simulink model "kalman"  (R2017a)
settings: Solver=VariableStepAuto  StartTime=0  StopTime=65  RelTol=1e-5
undefined symbols (not defined in the file): Discrete, Time
libraries: dspfdesign x3, ctrlSharedLib x1
settings Model: Creator=13291  LastModifiedBy=13291
settings DataIOCC: ExternalInput=[t, u, c1, c2]  LoadExternalInput=on

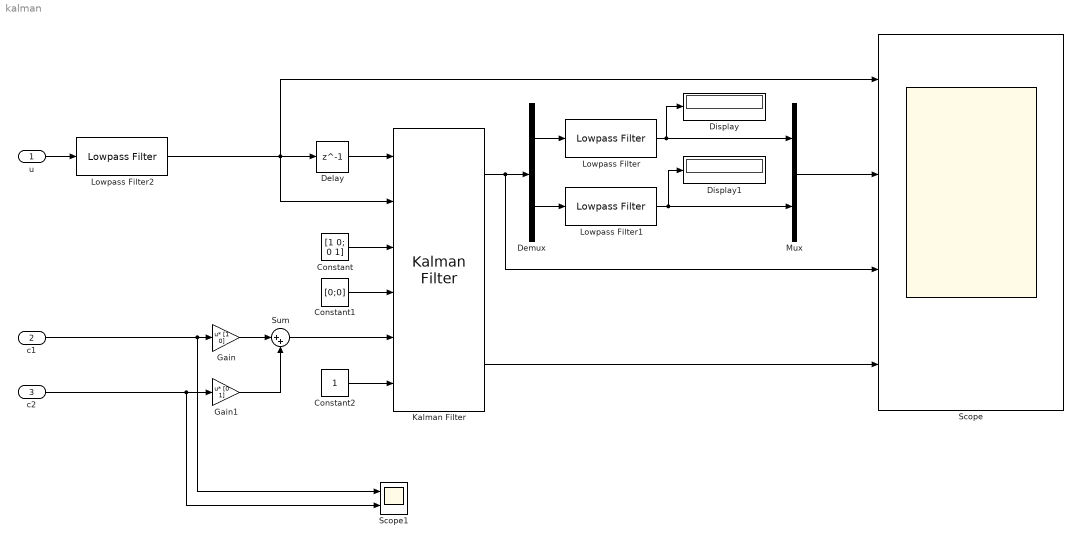
== system kalman ==
  u : Inport  PortDimensions=1  SampleTime=0.002
  c1 : Inport  Port=2  PortDimensions=1  SampleTime=0.002
  c2 : Inport  Port=3  PortDimensions=1  SampleTime=0.002
  Constant : Constant  Value=[1 0; 0 1]  VectorParams1D=off
  Constant1 : Constant  Value=[0;0]  VectorParams1D=off  LockScale=on
  Constant2 : Constant
  Delay : Delay  DelayLength=1
  Demux : Demux  Outputs=2
  Display : Display
  Display1 : Display
  Gain : Gain  Gain=[1 0]  Multiplication=Matrix(u*K)
  Gain1 : Gain  Gain=[0 1]  Multiplication=Matrix(u*K)
  Kalman Filter : ctrlSharedLib/Kalman Filter  TimeDomain=Discrete-Time  UseCurrentEstimator=on  ModelSource=Input port  ModelSourceVariable=ss(0.95,1,1,0,1)  A=0.95  B=1  C=1  D=0  NumberOfStates=2  NumberOfInputs=1  NumberOfOutputs=1  InitialEstimateSource=Dialog  X0=0  P0=10  UseK=off  UseGH=off  NumberOfProcessNoiseInputs=1  G=1  TimeInvariantG=on  H=0  TimeInvariantH=on  Q=1e2  TimeInvariantQ=on  R=1e2  TimeInvariantR=on  N=[0.5e2;0.5e2]  TimeInvariantN=on  AddInputPort=on  AddEnablePort=off  OutputEstimatedY=on  OutputP=on  Ts=0.002
  Lowpass Filter : dspfdesign/Lowpass Filter  FilterType=FIR  DesignForMinimumOrder=on  FilterOrder=50  PassbandFrequency=0.1  StopbandFrequency=0.5  PassbandRipple=0.1  StopbandAttenuation=80  InheritSampleRate=off  SampleRate=1/0.002  SimulateUsing=Interpreted execution  roundingMode=Floor  coeffsDataTypeStr=fixdt(1,16)
  Lowpass Filter1 : dspfdesign/Lowpass Filter  FilterType=FIR  DesignForMinimumOrder=on  FilterOrder=50  PassbandFrequency=0.1  StopbandFrequency=0.5  PassbandRipple=0.1  StopbandAttenuation=80  InheritSampleRate=off  SampleRate=1/0.002  SimulateUsing=Interpreted execution  roundingMode=Floor  coeffsDataTypeStr=fixdt(1,16)
  Lowpass Filter2 : dspfdesign/Lowpass Filter  FilterType=FIR  DesignForMinimumOrder=on  FilterOrder=50  PassbandFrequency=30  StopbandFrequency=40  PassbandRipple=0.1  StopbandAttenuation=80  InheritSampleRate=off  SampleRate=1/0.002  SimulateUsing=Interpreted execution  roundingMode=Floor  coeffsDataTypeStr=fixdt(1,16)
  Mux : Mux  Inputs=2
  Scope : Scope  NumInputPorts=4
  Scope1 : Scope  NumInputPorts=2
  Sum : Sum  Inputs=|++
  wires:
  Delay/1 -> Kalman Filter/1
  u/1 -> Lowpass Filter2/1
  Constant/1 -> Kalman Filter/3
  Constant1/1 -> Kalman Filter/4
  Gain/1 -> Sum/1
  Gain1/1 -> Sum/2
  Sum/1 -> Kalman Filter/5
  Constant2/1 -> Kalman Filter/6
  Kalman Filter/3 -> Scope/4
  Kalman Filter/1 -> Scope/3, Demux/1
  Demux/1 -> Lowpass Filter/1
  Lowpass Filter/1 -> Display/1, Mux/1
  Demux/2 -> Lowpass Filter1/1
  Lowpass Filter1/1 -> Display1/1, Mux/2
  Mux/1 -> Scope/2
  Lowpass Filter2/1 -> Scope/1, Kalman Filter/2, Delay/1
  c1/1 -> Scope1/1, Gain/1
  c2/1 -> Scope1/2, Gain1/1
